simulink model "Speedmeter2"  (R2019b)
settings: Solver=FixedStepDiscrete  StartTime=0  StopTime=10  FixedStep=STEP_TIME  RelTol=1e-3  EnableMultiTasking=on
undefined symbols (not defined in the file or in its folder): Const16_0, Const16_2, Const16_210, Const16_340, Const16_350, Const16_4, Const8_0, Const8_1, Const8_2, Const8_4, ConstFL_00879, ConstFL_01, ConstFL_03516, ConstFL_1_6093, STEP_TIME
libraries: simulink x1
(part 2 of 2)

== system Speedmeter2/SWC_SpeedMeter/SWC_SpeedMeter/Spd_Pointer/PointerAngleCalculation/SwitchCaseActionSubsystem2 ==
  VH_usAvgVehicleSpeed : Inport  PortDimensions=1  SampleTime=STEP_TIME
  IH_usSMV : Inport  Port=2  OutMin=0  OutMax=4095  SampleTime=STEP_TIME
  IH_usSMD : Inport  Port=3  OutMin=0  OutMax=4095  SampleTime=STEP_TIME
  Action Port : ActionPort  ActionPortLabel=else
  Lookup Table Dynamic : simulink/Lookup Tables/Lookup Table Dynamic  LookUpMeth=Interpolation-Use End Values  OutDataType=fixdt(0,16,0.1,0)  OutScaling=[]  OutDataTypeStr=Inherit: Inherit via back propagation  DoSatur=off
      settings: SourceProductName=Simulink
  PointerAngle : Outport  SampleTime=STEP_TIME  VectorParamsAs1DForOutWhenUnconnected=off
  wires:
  VH_usAvgVehicleSpeed/1 -> Lookup Table Dynamic/1
  IH_usSMV/1 -> Lookup Table Dynamic/2
  Lookup Table Dynamic/1 -> PointerAngle/1
  IH_usSMD/1 -> Lookup Table Dynamic/3

== system Speedmeter2/SWC_SpeedMeter/SWC_SpeedMeter/Spd_Pointer/PointerAngleCalculation/SwitchCaseActionSubsystem3 ==
  VH_usAvgVehicleSpeed : Inport  SampleTime=STEP_TIME
  IH_usSMV : Inport  Port=2  OutMin=0  OutMax=4095  SampleTime=STEP_TIME
  IH_usSMD : Inport  Port=3  OutMin=0  OutMax=4095  SampleTime=STEP_TIME
  Action Port : ActionPort  ActionPortLabel=if(u1 == 1)
  Divide : Product  Inputs=*/  OutDataTypeStr=Inherit: Inherit via back propagation  SaturateOnIntegerOverflow=on  InputSameDT=on
  Multiply3 : Product  OutDataTypeStr=Inherit: Inherit via back propagation  InputSameDT=on
  Selector : Selector  IndexMode=Zero-based  InputPortWidth=13  IndexOptions=Index vector (dialog)  Indices=[11]  OutputSizes=1
  Selector1 : Selector  IndexMode=Zero-based  InputPortWidth=13  IndexOptions=Index vector (dialog)  Indices=[12]  OutputSizes=1
  Selector2 : Selector  IndexMode=Zero-based  InputPortWidth=13  IndexOptions=Index vector (dialog)  Indices=[12]  OutputSizes=1
  Selector3 : Selector  IndexMode=Zero-based  InputPortWidth=13  IndexOptions=Index vector (dialog)  Indices=[11]  OutputSizes=1
  Subtract1 : Sum  Inputs=+-  OutDataTypeStr=Inherit: Inherit via back propagation  InputSameDT=on
  Subtract2 : Sum  Inputs=+-  InputSameDT=on  OutDataTypeStr=Inherit: Same as first input
  Subtract3 : Sum  Inputs=+-  OutDataTypeStr=Inherit: Inherit via back propagation  InputSameDT=on
  Subtract4 : Sum  OutDataTypeStr=Inherit: Inherit via back propagation  InputSameDT=on
  PointerAngle : Outport  SampleTime=STEP_TIME  VectorParamsAs1DForOutWhenUnconnected=off
  wires:
  Subtract4/1 -> PointerAngle/1
  VH_usAvgVehicleSpeed/1 -> Subtract1/1
  Subtract1/1 -> Divide/1
  Selector3/1 -> Subtract4/2, Subtract2/2
  Selector/1 -> Subtract3/2, Subtract1/2
  Multiply3/1 -> Subtract4/1
  Selector2/1 -> Subtract2/1
  Divide/1 -> Multiply3/2
  Subtract2/1 -> Multiply3/1
  IH_usSMV/1 -> Selector/1, Selector1/1
  IH_usSMD/1 -> Selector3/1, Selector2/1
  Subtract3/1 -> Divide/2
  Selector1/1 -> Subtract3/1

== stateflow chart Speedmeter2/SWC_SpeedMeter/SWC_SpeedMeter/Spd_Common/HeapSort ==
  state K1  = HeapSort(InitPos, Len, N) [function]
    note: /*Perform Heapsort sorting for Key array K
        | Input Argument:
        | InitPos:Start index position for sorting
        | Len:	Len the of the values in array to be sorted
        | N:	Key array
        | PriOrderArr:	2-D array
        |
        | Output Argument:
        | K1= Sorted Key array;
        | HeapifyOut = Sorted 2-D array
        | Flag = Contains status of sorting algorithm
        | */
    (default) -> (junction 2826)
    (junction 2826) -> (junction 2827) [order 1] : [Len <= 1]
        | {Flag = FALSE;}
    (junction 2826) -> (junction 2828) [order 2]
    (junction 2827) -> (junction 2833)
    (junction 2828) -> (junction 2829) [order 1] : [Len > R_MD_AD2ARNDCARMAX]
    (junction 2828) -> (junction 2830) [order 2]
    (junction 2829) -> (junction 2831) : {Len = R_MD_AD2ARNDCARMAX;}
    (junction 2831) -> (junction 2830)
    (junction 2830) -> (junction 2832)
    (junction 2832) -> (junction 2833) [order 1] : [InitPos < 0 ]
        | {Flag=FALSE;}
    (junction 2832) -> (junction 2834) [order 2]
    (junction 2833) -> (junction 2835)
    (junction 2834) -> (junction 2835) [order 1] : [((InitPos + Len - 1) >= R_MD_AD2ARNDCARMAX)]
        | {Flag=FALSE;}
    (junction 2834) -> (junction 2837) [order 2] : {
        | LNode = Len -1+InitPos ;
        | RNode = InitPos;}
    (junction 2835) -> (junction 2839)
    (junction 2836) -> (junction 2837)
    (junction 2864) -> (junction 2836)
    (junction 2837) -> (junction 2838)
    (junction 2838) -> (junction 2839) [order 2] : {Flag=TRUE;}
    (junction 2838) -> (junction 2841) [order 1] : [RNode <LNode]
        | {
        | PNode = (((LNode-1 - RNode ) )/2) + RNode;
        | MNode = PNode;
        | }
    (junction 2839) -> (junction 2853)
    (junction 2840) -> (junction 2841)
    (junction 2841) -> (junction 2843) : {CLNode = (2*PNode + 1) - RNode;
        | CRNode = (2*PNode + 2) - RNode;}
    (junction 2861) -> (junction 2840)
    (junction 2843) -> (junction 2842) [order 1] : [N[PNode] <= N[CLNode]]
    (junction 2843) -> (junction 2844) [order 2] : {select_val = N[CLNode];
        | select_node = CLNode;}
    (junction 2842) -> (junction 2845) : {select_val = N[PNode];
        | select_node = PNode;}
    (junction 2845) -> (junction 2844)
    (junction 2844) -> (junction 2846)
    (junction 2846) -> (junction 2847) [order 1] : [(CRNode <= LNode) ]
    (junction 2847) -> (junction 2848) [order 1] : [(select_val > N[CRNode])]
    (junction 2846) -> (junction 2849) [order 2] : {CRNode=0;}
    (junction 2847) -> (junction 2850) [order 2]
    (junction 2848) -> (junction 2851) : {select_val = N[CRNode];
        | select_node = CRNode;}
    (junction 2850) -> (junction 2849)
    (junction 2851) -> (junction 2850)
    (junction 2849) -> (junction 2854)
    (junction 2854) -> (junction 2855) [order 2]
    (junction 2855) -> (junction 2852) [order 2]
    (junction 2852) -> (junction 2853) [order 2] : {Flag=FALSE;}
    (junction 2854) -> (junction 2856) [order 1] : [N[select_node]==N[PNode]]
        | {MNode--;
        | PNode = MNode;}
    (junction 2855) -> (junction 2857) [order 1] : [N[select_node]==N[CLNode]]
        | {work_val = N[PNode];
        | N[PNode] = N[CLNode];
        | N[CLNode] = work_val;
        | PNode = CLNode;
        | }
    (junction 2852) -> (junction 2858) [order 1] : [CRNode>=2 && N[select_node]==N[CRNode]]
        | {work_val = N[PNode];
        | N[PNode] = N[CRNode];
        | N[CRNode] = work_val;
        | PNode = CRNode;
        | }
    (junction 2853) -> (junction 2866) : {  K1[0]=N[0];
        | K1[1]=N[1];
        | K1[2]=N[2];
        | K1[3]=N[3];
        | K1[4]=N[4];
        | K1[5]=N[5];
        | K1[6]=N[6];
        | K1[7]=N[7];
        | K1[8]=N[8];
        | K1[9]=N[9];
        | K1[10]=N[10];
        | K1[11]=N[11];
        | K1[12]=N[12];
        | K1[13]=N[13];
        | K1[14]=N[14];
        | K1[15]=N[15];}
    (junction 2856) -> (junction 2857)
    (junction 2858) -> (junction 2857)
    (junction 2857) -> (junction 2860) : {work_CLNode = (2*PNode + 1) - RNode;
        | }
    (junction 2860) -> (junction 2859) [order 1] : [work_CLNode > LNode]
    (junction 2859) -> (junction 2863) : {MNode--;
        | PNode = MNode;}
    (junction 2860) -> (junction 2862) [order 2]
    (junction 2862) -> (junction 2861) [order 2]
    (junction 2863) -> (junction 2862)
    (junction 2862) -> (junction 2865) [order 1] : [MNode < RNode]
    (junction 2865) -> (junction 2864) : {RNode++;}
  (default) -> (junction 1643) : {
      | K1Arr = yLineArr; /*Create array K1 with yline values*/
      | K = HeapSort(0, 16, K1Arr);/* Sort K1 using Heapsort*/
      | }
  data: InitPos function_input uint8; Len function_input uint8 size=1; N function_input fixdt(0,16,0.01,0) size=16; K1 function_output fixdt(0,16,0.01,0) size=16; FALSE constant boolean =0; TRUE constant boolean =1; CLNode local int8; CRNode local int8; LNode local int8; MNode local int8; PNode local int8; RNode local int8; work_val local fixdt(0,16,0.01,0); select_node local int8; select_val local fixdt(0,16,0.01,0); R_MD_AD2ARNDCARMAX constant uint8 =16; yLineArr input fixdt(0,16,0.01,0) size=16; work_CLNode local int8; Flag local int8; K output fixdt(0,16,0.01,0) size=16; K1Arr local fixdt(0,16,0.01,0) size=16
  data InitPos settings: description=$TL$ type=UInt8; $TL$
  data Len settings: description=$TL$ type=UInt8; $TL$
  data N settings: description=$TL$ type=UInt16; $TL$
  data K1 settings: description=$TL$ type=UInt16; $TL$
  data FALSE settings: description=$TL$ type=UInt8; $TL$
  data TRUE settings: description=$TL$ type=UInt8; $TL$
  data CLNode settings: description=$TL$ type=UInt16; $TL$
  data CRNode settings: description=$TL$ type=UInt16; $TL$
  data LNode settings: description=$TL$ type=UInt16; $TL$
  data MNode settings: description=$TL$ type=Int8; $TL$
  data PNode settings: description=$TL$ type=UInt16; $TL$
  data RNode settings: description=$TL$ type=UInt8; $TL$
  data work_val settings: description=$TL$ type=UInt16; $TL$
  data select_node settings: description=$TL$ type=UInt8; $TL$
  data select_val settings: description=$TL$ type=UInt16; $TL$
  data R_MD_AD2ARNDCARMAX settings: description=$TL$ type=UInt8; $TL$
  data yLineArr settings: description=$TL$ type=UInt16; $TL$
  data work_CLNode settings: description=$TL$ type=UInt16; $TL$
  data K settings: description=$TL$ type=UInt16; $TL$
